simulink model "noise_filter_16_bit"  (R2016b)
settings: Solver=FixedStepDiscrete  StartTime=0.0  StopTime=50  RelTol=1e-3
undefined symbols (not defined in the file or in its folder): Fs, get, Radix
libraries: dspsnks4 x6, hdlsllib x4, dspxfrm3 x4, simulink x1, dspsrcs4 x1, dspsigops x1
settings Model: DataTypeOverride=Off  Creator=mw  LastModifiedBy=jake
settings DataIOCC: SaveOutput=off  SaveTime=off
settings OptimizationCC: BlockReduction=off  ConditionallyExecuteInputs=off  DefaultParameterBehavior=Inlined
settings DebuggingCC: AlgebraicLoopMsg=error  SingleTaskRateTransMsg=error  StrictBusMsg=ErrorOnBusTreatedAsVector
settings HardwareCC: ProdBitPerPointer=32  ProdBitPerSizeT=32  ProdBitPerPtrDiffT=32  ProdLargestAtomicFloat=None  ProdIntDivRoundTo=Undefined  ProdEndianess=Unspecified  ProdWordSize=32  ProdHWDeviceType=ASIC/FPGA->ASIC/FPGA  ProdEqTarget=off
settings GRTTargetCC: TargetLangStandard=C89/C90 (ANSI)

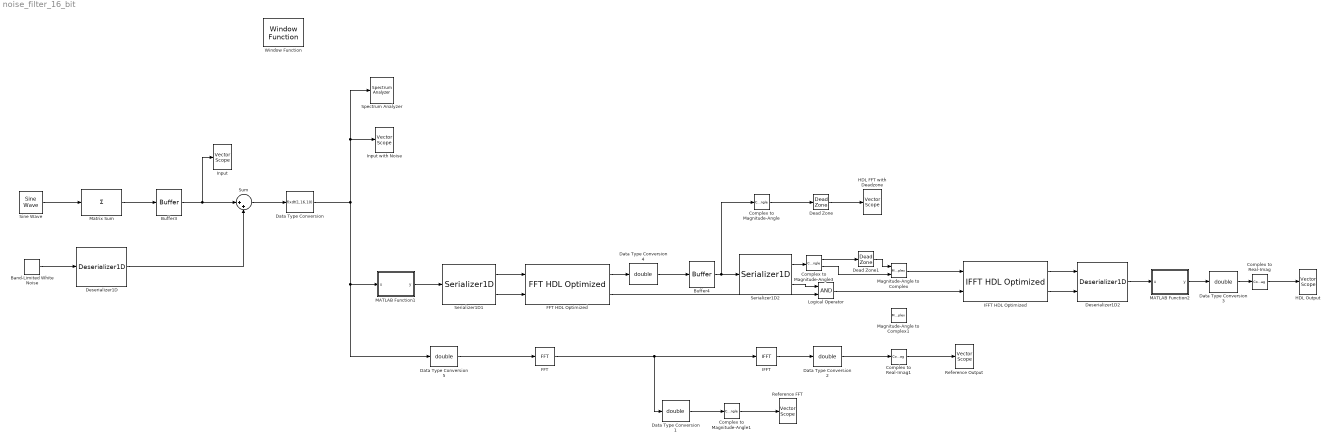
== system noise_filter_16_bit ==
  Band-Limited White Noise : simulink/Sources/Band-Limited White Noise  Cov=0.04  Ts=1 / 1024  seed=[23341]
  Buffer3 : Buffer  N=1024  TreatMby1Signals=One channel  OutputFrames=off
  Buffer4 : Buffer  N=1024  TreatMby1Signals=One channel  OutputFrames=off
  Complex to Magnitude-Angle : ComplexToMagnitudeAngle  Output=Magnitude
  Complex to Magnitude-Angle1 : ComplexToMagnitudeAngle  Output=Magnitude
  Complex to Magnitude-Angle3 : ComplexToMagnitudeAngle
  Complex to Real-Imag : ComplexToRealImag  Output=Real
  Complex to Real-Imag1 : ComplexToRealImag  Output=Real
  Data Type Conversion : DataTypeConversion  OutDataTypeStr=fixdt(1,16,10)
  Data Type Conversion1 : DataTypeConversion  OutDataTypeStr=double  RndMeth=Nearest
  Data Type Conversion2 : DataTypeConversion  OutDataTypeStr=double  RndMeth=Nearest
  Data Type Conversion3 : DataTypeConversion  OutDataTypeStr=double  RndMeth=Nearest
  Data Type Conversion4 : DataTypeConversion  OutDataTypeStr=double
  Data Type Conversion5 : DataTypeConversion  OutDataTypeStr=double
  Dead Zone : DeadZone  LowerValue=0  UpperValue=10^3  SaturateOnIntegerOverflow=on
  Dead Zone1 : DeadZone  LowerValue=0  UpperValue=4*10^2  SaturateOnIntegerOverflow=on
  Deserializer1D : hdlsllib/HDL Operations/Deserializer1D  Ratio=1024  IdleCycles=0  InitialCondition=0  startIn=off  validIn=off  validOut=off  inputDataDimensions=-1  inputSampleTime=-1  inputSignalType=auto
  Deserializer1D2 : hdlsllib/HDL Operations/Deserializer1D  Ratio=16  IdleCycles=0  InitialCondition=0  startIn=off  validIn=on  validOut=off  inputDataDimensions=-1  inputSampleTime=-1  inputSignalType=auto
  FFT : dspxfrm3/FFT  FFTImplementation=Radix-2  CompMethod=Table lookup  TableOpt=NEW  TableOptActive=Speed  BitRevOrder=off  Normalize=off  InheritFFTLength=off  FFTLength=1024  WrapInput=off  roundingMode=Nearest  overflowMode=off  firstCoeffDataTypeStr=Inherit: Same word length as input  firstCoeffLastDataTypeStr=Inherit: Same word length as input  outputMin=[]  outputMax=[]
      settings: LockScale=on
  FFT HDL Optimized : dspxfrm3/FFT HDL Optimized  Architecture=Streaming Radix 2^2  ComplexMultiplication=Use 3 multipliers and 5 adders  BitReversedOutput=off  BitReversedInput=on  Normalize=off  FFTLength=1024  SimulateUsing=Code generation  RoundingMethod=Floor  ResetInputPort=off  StartOutputPort=off  EndOutputPort=off
  HDL FFT with Deadzone : dspsnks4/Vector Scope  ScopeProperties=on  Domain=Frequency  HorizSpan=1  DisplayProperties=off  AxisGrid=on  Memory=off  FrameNumber=on  AxisLegend=off  AxisZoom=off  OpenScopeAtSimStart=on  OpenScopeImmediately=off  FigPos=get(0,'defaultfigureposition')  AxisProperties=off  XUnits=Hertz  XRange=[-Fs/2...Fs/2]  InheritXIncr=on  XIncr=1/4096  XLabel=Time  XLimit=Auto  XMin=-50  XMax=50  XStart=0  YUnits=dB  YLabel=Amplitude  LineProperties=off  XAxisParamsVer=6.9
      settings: YMin=-50  YMax=50
  HDL Output : dspsnks4/Vector Scope  ScopeProperties=on  Domain=Time  HorizSpan=1  DisplayProperties=off  AxisGrid=on  Memory=off  FrameNumber=on  AxisLegend=off  AxisZoom=off  OpenScopeAtSimStart=on  OpenScopeImmediately=off  FigPos=get(0,'defaultfigureposition')  AxisProperties=off  XUnits=Hertz  XRange=[0...Fs/2]  InheritXIncr=on  XIncr=1  XLabel=Time  XLimit=Auto  XMin=0  XMax=15  XStart=0  YUnits=dB  YLabel=Amplitude  LineProperties=off  XAxisParamsVer=6.9
      settings: YMin=-40  YMax=40
  IFFT : dspxfrm3/IFFT  FFTImplementation=Radix-2  CompMethod=Table lookup  TableOpt=NEW  TableOptActive=Speed  BitRevOrder=off  cs_in=off  Normalize=on  InheritFFTLength=off  FFTLength=1024  WrapInput=on  mode=Complex  outSamplingMode=Sample based  roundingMode=Nearest  overflowMode=off  firstCoeffDataTypeStr=Inherit: Same word length as input  firstCoeffLastDataTypeStr=Inherit: Same word length as input  outputMin=[]  outputMax=[]
  IFFT HDL Optimized : dspxfrm3/IFFT HDL Optimized  Architecture=Streaming Radix 2^2  ComplexMultiplication=Use 3 multipliers and 5 adders  BitReversedOutput=on  BitReversedInput=off  Normalize=on  FFTLength=1024  SimulateUsing=Code generation  RoundingMethod=Floor  ResetInputPort=off  StartOutputPort=off  EndOutputPort=off
  Input : dspsnks4/Vector Scope  ScopeProperties=on  Domain=Time  HorizSpan=1  DisplayProperties=off  AxisGrid=on  Memory=off  FrameNumber=on  AxisLegend=off  AxisZoom=off  OpenScopeAtSimStart=on  OpenScopeImmediately=off  FigPos=get(0,'defaultfigureposition')  AxisProperties=off  XUnits=Hertz  XRange=[0...Fs/2]  InheritXIncr=on  XIncr=1  XLabel=Time  XLimit=Auto  XMin=0  XMax=1  XStart=0  YUnits=dB  YLabel=Amplitude  LineProperties=off  XAxisParamsVer=6.9
      settings: YMin=-40  YMax=40
  Input with Noise : dspsnks4/Vector Scope  ScopeProperties=on  Domain=Time  HorizSpan=1  DisplayProperties=off  AxisGrid=on  Memory=off  FrameNumber=on  AxisLegend=off  AxisZoom=off  OpenScopeAtSimStart=on  OpenScopeImmediately=off  FigPos=get(0,'defaultfigureposition')  AxisProperties=off  XUnits=Hertz  XRange=[0...Fs/2]  InheritXIncr=on  XIncr=1  XLabel=Time  XLimit=Auto  XMin=0  XMax=1  XStart=0  YUnits=dB  YLabel=Amplitude  LineProperties=off  XAxisParamsVer=6.9
      settings: YMin=-40  YMax=40
  Logical Operator : Logic  AllPortsSameDT=off  OutDataTypeStr=boolean
  MATLAB Function1 : MATLAB Function  TreatAsAtomicUnit=on
  MATLAB Function2 : MATLAB Function  TreatAsAtomicUnit=on
  Magnitude-Angle to Complex : MagnitudeAngleToComplex
  Magnitude-Angle to Complex1 : MagnitudeAngleToComplex
  Matrix Sum : Sum  Inputs=+  CollapseMode=Specified dimension  CollapseDim=2
  Reference FFT : dspsnks4/Vector Scope  ScopeProperties=on  Domain=Frequency  HorizSpan=1  DisplayProperties=off  AxisGrid=on  Memory=off  FrameNumber=on  AxisLegend=off  AxisZoom=off  OpenScopeAtSimStart=on  OpenScopeImmediately=off  FigPos=get(0,'defaultfigureposition')  AxisProperties=off  XUnits=Hertz  XRange=[-Fs/2...Fs/2]  InheritXIncr=on  XIncr=1/4096  XLabel=Time  XLimit=Auto  XMin=-50  XMax=50  XStart=0  YUnits=dB  YLabel=Amplitude  LineProperties=off  XAxisParamsVer=6.9
      settings: YMin=-50  YMax=50
  Reference Output : dspsnks4/Vector Scope  ScopeProperties=on  Domain=Time  HorizSpan=1  DisplayProperties=off  AxisGrid=on  Memory=off  FrameNumber=on  AxisLegend=off  AxisZoom=off  OpenScopeAtSimStart=on  OpenScopeImmediately=off  FigPos=get(0,'defaultfigureposition')  AxisProperties=off  XUnits=Hertz  XRange=[0...Fs/2]  InheritXIncr=on  XIncr=1  XLabel=Time  XLimit=Auto  XMin=0  XMax=15  XStart=0  YUnits=dB  YLabel=Amplitude  LineProperties=off  XAxisParamsVer=6.9
      settings: YMin=-40  YMax=40
  Serializer1D1 : hdlsllib/HDL Operations/Serializer1D  Ratio=16  IdleCycles=0  validIn=off  startOut=off  validOut=on  inputDataDimensions=-1  inputSampleTime=-1  inputSignalType=auto
  Serializer1D2 : hdlsllib/HDL Operations/Serializer1D  Ratio=16  IdleCycles=0  validIn=off  startOut=off  validOut=on  inputDataDimensions=-1  inputSampleTime=-1  inputSignalType=auto
  Sine Wave : dspsrcs4/Sine Wave  Amplitude=[4,8,8,4]  Frequency=[5,10,20,30]  Phase=[0,0.2,-pi/2, 3]  SampleMode=Discrete  OutComplex=Real  CompMethod=Trigonometric fcn  TableSize=Speed  SampleTime=1 / (16*64)  SamplesPerFrame=64  ResetState=Restart at time zero  OutputFrames=off  dataType=double  wordLen=16  udDataType=sfix(16)  fracBitsMode=Best precision  numFracBits=15  OutDataTypeStr=double  LastOutDataTypeStr=double
  Spectrum Analyzer : SpectrumAnalyzer
  Sum : Sum  Inputs=|++
  Window Function : dspsigops/Window Function  winmode=Apply window to input  wintype=Hamming  sampmode=Continuous  samptime=1  N=64  Rs=50  beta=10  winsamp=Symmetric  UserWindow=hamming  OptParams=off  UserParams={'symmetric'}  dataType=double  isSigned=on  wordLen=16  udDataType=sfix(16)  fracBitsMode=Best precision  numFracBits=15  outputMode=Binary point scaling  outputWordLength=16  outputFracLength=10  roundingMode=Floor  overflowMode=off  numSidelobes=4  sidelobeLevel=-30
  wires:
  Sine Wave/1 -> Matrix Sum/1
  Complex to Real-Imag/1 -> HDL Output/1
  MATLAB Function1/1(y) -> Serializer1D1/1
  Deserializer1D2/1 -> MATLAB Function2/1(u)
  Buffer4/1 -> Complex to Magnitude-Angle/1, Serializer1D2/1
  IFFT HDL Optimized/2 -> Deserializer1D2/2
  Serializer1D1/1 -> FFT HDL Optimized/1
  MATLAB Function2/1(y) -> Data Type Conversion3/1
  FFT HDL Optimized/2 -> Logical Operator/2
  FFT/1 -> Data Type Conversion1/1, IFFT/1
  Complex to Real-Imag1/1 -> Reference Output/1
  IFFT/1 -> Data Type Conversion2/1
  Complex to Magnitude-Angle1/1 -> Reference FFT/1
  Band-Limited White Noise/1 -> Deserializer1D/1
  Data Type Conversion1/1 -> Complex to Magnitude-Angle1/1
  Data Type Conversion2/1 -> Complex to Real-Imag1/1
  Data Type Conversion3/1 -> Complex to Real-Imag/1
  Serializer1D1/2 -> FFT HDL Optimized/2
  Logical Operator/1 -> IFFT HDL Optimized/2
  Complex to Magnitude-Angle/1 -> Dead Zone/1
  Dead Zone/1 -> HDL FFT with Deadzone/1
  Complex to Magnitude-Angle3/1 -> Dead Zone1/1
  Dead Zone1/1 -> Magnitude-Angle to Complex/1
  Serializer1D2/2 -> Logical Operator/1
  Magnitude-Angle to Complex/1 -> IFFT HDL Optimized/1
  IFFT HDL Optimized/1 -> Deserializer1D2/1
  Complex to Magnitude-Angle3/2 -> Magnitude-Angle to Complex/2
  Matrix Sum/1 -> Buffer3/1
  Data Type Conversion5/1 -> FFT/1
  FFT HDL Optimized/1 -> Data Type Conversion4/1
  Data Type Conversion4/1 -> Buffer4/1
  Serializer1D2/1 -> Complex to Magnitude-Angle3/1
  Data Type Conversion/1 -> Input with Noise/1, Spectrum Analyzer/1, Data Type Conversion5/1, MATLAB Function1/1(u)
  Buffer3/1 -> Input/1, Sum/1
  Sum/1 -> Data Type Conversion/1
  Deserializer1D/1 -> Sum/2

== matlab function noise_filter_16_bit/MATLAB Function1 ==
  data: u input; y output
function y = bit_reverse(u)
    coder.varsize('bit-reverse', [1024 1]);
    u = bitrevorder(u);
y = u;
end

== matlab function noise_filter_16_bit/MATLAB Function2 ==
  data: u input; y output
function y = bit_reverse(u)
    coder.varsize('bit-reverse', [1024 1]);
    u = bitrevorder(u);
y = u;
end
